simulink model "Formation"  (R2019b)
settings: Solver=FixedStepAuto  StartTime=0.0  StopTime=tf  FixedStep=Ts  RelTol=1e-3
values from neighbouring files (symbols this model uses):
  n = size(L,1)    [Formation_Design.m]    (also in Sim_Parameters.m = 4; anim.m = size(z_tt,1))
  z_0_t = [-2    2    0 ... (first row only)    [Formation_Design.m]
libraries: eeGeneralControl x1
settings Model: Creator=AMIN  LastModifiedBy=AMIN
settings DataIOCC: SaveFormat=Array  ReturnWorkspaceOutputs=off
settings SFSimCC: CustomCodeUndefinedFunction=UseInterfaceOnly

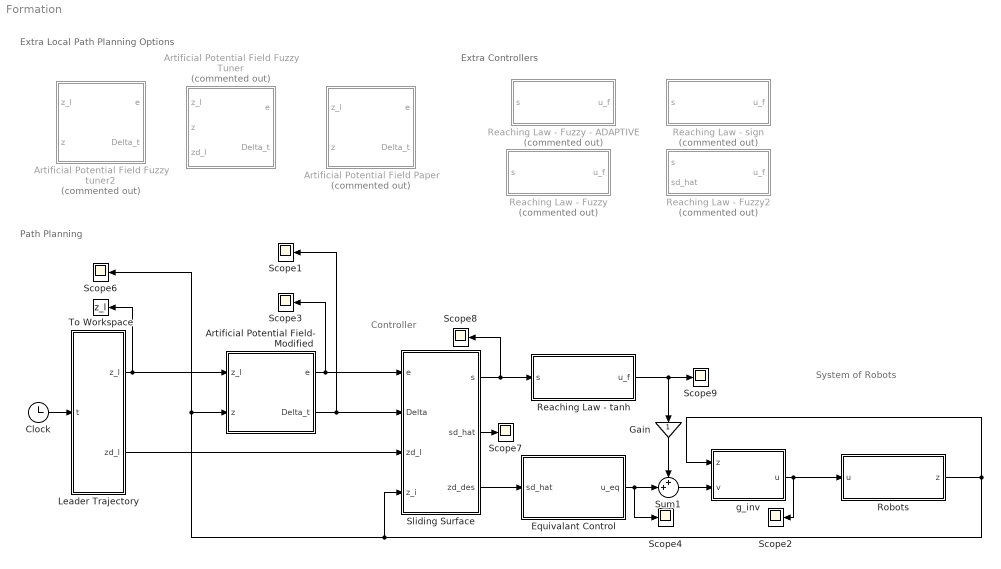
== system Formation ==
  note: Extra Local Path Planning Options
  note: Extra Controllers
  note: System of Robots
  note: Controller
  note: Path Planning
  Artificial Potential Field Fuzzy Tuner : Subsystem  Commented=on
  Artificial Potential Field Fuzzy tuner2 : Subsystem  Commented=on
  Artificial Potential Field Paper : Subsystem  Commented=on
  Artificial Potential Field- Modified : Subsystem
  Clock : Clock
  Equivalant Control : MATLAB Function  TreatAsAtomicUnit=on
  Gain : Gain
  Leader Trajectory : MATLAB Function  TreatAsAtomicUnit=on
  Reaching Law - Fuzzy : Subsystem  Commented=on
  "Reaching Law - Fuzzy - ADAPTIVE " : Subsystem  Commented=on
  Reaching Law - Fuzzy2 : Subsystem  Commented=on
  Reaching Law - sign : Subsystem  Commented=on
  Reaching Law - tanh : Subsystem
  Robots : Subsystem
  Scope{1..4,6..9} (8 alike) : Scope
  Sliding Surface : Subsystem
  Sum1 : Sum  Inputs=++|
  To Workspace : ToWorkspace  VariableName=z_l  SampleTime=-1
  g_inv : MATLAB Function  TreatAsAtomicUnit=on
  wires:
  Sum1/1 -> g_inv/2(v)
  Robots/1(z) -> g_inv/1(z), Sliding Surface/4(z_i), Artificial Potential Field- Modified/2(z), Scope6/1
  Clock/1 -> Leader Trajectory/1(t)
  Leader Trajectory/1(z_l) -> To Workspace/1, Artificial Potential Field- Modified/1(z_l)
  Sliding Surface/1(s) -> Reaching Law - tanh/1(s), Scope8/1
  Equivalant Control/1(u_eq) -> Sum1/2, Scope4/1
  Gain/1 -> Sum1/1
  Leader Trajectory/2(zd_l) -> Sliding Surface/3(zd_l)
  Sliding Surface/3(zd_des) -> Equivalant Control/1(sd_hat)
  Sliding Surface/2(sd_hat) -> Scope7/1
  g_inv/1(u) -> Robots/1(u), Scope2/1
  Artificial Potential Field- Modified/1(e) -> Scope3/1, Sliding Surface/1(e)
  Artificial Potential Field- Modified/2(Delta_t) -> Scope1/1, Sliding Surface/2(Delta)
  Reaching Law - tanh/1(u_f) -> Gain/1, Scope9/1

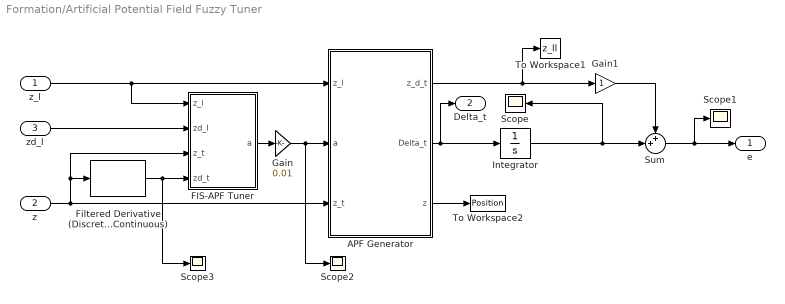
== system Formation/Artificial Potential Field Fuzzy Tuner ==
  z_l : Inport
  z : Inport  Port=2
  zd_l : Inport  Port=3
  APF Generator : MATLAB Function  TreatAsAtomicUnit=on
  FIS-APF Tuner : MATLAB Function  TreatAsAtomicUnit=on
  Filtered Derivative (Discrete or Continuous) : eeGeneralControl/Filtered Derivative (Discrete or Continuous)  K=1  T=100  B=inf  A=-inf  minRatio=10  Ts=-1
      settings: SourceProductName=Simscape Electrical  SourceProductBaseCode=PS
  Gain : Gain  Gain=0.01
  Gain1 : Gain
  Integrator : Integrator
  Scope{,1..3} (4 alike) : Scope
  Sum : Sum  Inputs=++|
  To Workspace1 : ToWorkspace  VariableName=z_ll  SaveFormat=Structure With Time  SampleTime=-1
  To Workspace2 : ToWorkspace  VariableName=Position  SaveFormat=Structure With Time  SampleTime=-1
  e : Outport  VectorParamsAs1DForOutWhenUnconnected=off
  Delta_t : Outport  Port=2  VectorParamsAs1DForOutWhenUnconnected=off
  wires:
  Sum/1 -> e/1, Scope1/1
  APF Generator/1(z_d_t) -> To Workspace1/1, Gain1/1
  Integrator/1 -> Scope/1, Sum/2
  APF Generator/2(Delta_t) -> Integrator/1, Delta_t/1
  Gain1/1 -> Sum/1
  FIS-APF Tuner/1(a) -> Gain/1
  APF Generator/3(z) -> To Workspace2/1
  Gain/1 -> APF Generator/2(a), Scope2/1
  z_l/1 -> FIS-APF Tuner/1(z_l), APF Generator/1(z_l)
  zd_l/1 -> FIS-APF Tuner/2(zd_l)
  z/1 -> APF Generator/3(z_t), Filtered Derivative (Discrete or Continuous)/1, FIS-APF Tuner/3(z_t)
  Filtered Derivative (Discrete or Continuous)/1 -> Scope3/1, FIS-APF Tuner/4(zd_t)

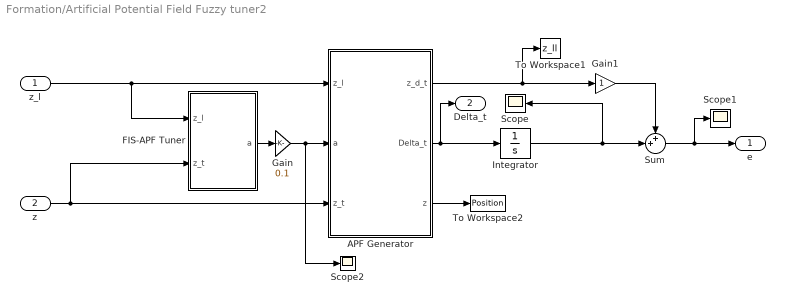
== system Formation/Artificial Potential Field Fuzzy tuner2 ==
  z_l : Inport
  z : Inport  Port=2
  APF Generator : MATLAB Function  TreatAsAtomicUnit=on
  FIS-APF Tuner : MATLAB Function  TreatAsAtomicUnit=on
  Gain : Gain  Gain=0.1
  Gain1 : Gain
  Integrator : Integrator
  Scope : Scope
  Scope1 : Scope
  Scope2 : Scope
  Sum : Sum  Inputs=++|
  To Workspace1 : ToWorkspace  VariableName=z_ll  SaveFormat=Structure With Time  SampleTime=-1
  To Workspace2 : ToWorkspace  VariableName=Position  SaveFormat=Structure With Time  SampleTime=-1
  e : Outport  VectorParamsAs1DForOutWhenUnconnected=off
  Delta_t : Outport  Port=2  VectorParamsAs1DForOutWhenUnconnected=off
  wires:
  Sum/1 -> e/1, Scope1/1
  APF Generator/1(z_d_t) -> To Workspace1/1, Gain1/1
  Integrator/1 -> Scope/1, Sum/2
  APF Generator/2(Delta_t) -> Integrator/1, Delta_t/1
  Gain1/1 -> Sum/1
  FIS-APF Tuner/1(a) -> Gain/1
  APF Generator/3(z) -> To Workspace2/1
  Gain/1 -> APF Generator/2(a), Scope2/1
  z_l/1 -> FIS-APF Tuner/1(z_l), APF Generator/1(z_l)
  z/1 -> APF Generator/3(z_t), FIS-APF Tuner/2(z_t)

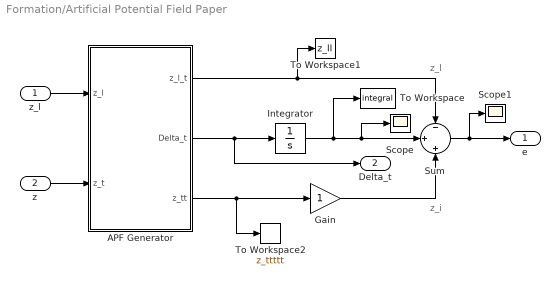
== system Formation/Artificial Potential Field Paper ==
  note: z_l
  note: z_i
  z_l : Inport
  z : Inport  Port=2
  APF Generator : MATLAB Function  TreatAsAtomicUnit=on
  Gain : Gain
  Integrator : Integrator
  Scope : Scope
  Scope1 : Scope
  Sum : Sum  Inputs=-|+|+
  To Workspace : ToWorkspace  VariableName=integral  SaveFormat=Structure With Time  SampleTime=-1
  To Workspace1 : ToWorkspace  VariableName=z_ll  SaveFormat=Structure With Time  SampleTime=-1
  To Workspace2 : ToWorkspace  VariableName=z_ttttt  SaveFormat=Structure With Time  SampleTime=-1
  e : Outport  VectorParamsAs1DForOutWhenUnconnected=off
  Delta_t : Outport  Port=2  VectorParamsAs1DForOutWhenUnconnected=off
  wires:
  APF Generator/2(Delta_t) -> Delta_t/1, Integrator/1
  z_l/1 -> APF Generator/1(z_l)
  z/1 -> APF Generator/2(z_t)
  Integrator/1 -> Scope/1, Sum/2, To Workspace/1
  APF Generator/1(z_l_t) -> To Workspace1/1, Sum/1
  APF Generator/3(z_tt) -> Gain/1, To Workspace2/1
  Sum/1 -> Scope1/1, e/1
  Gain/1 -> Sum/3

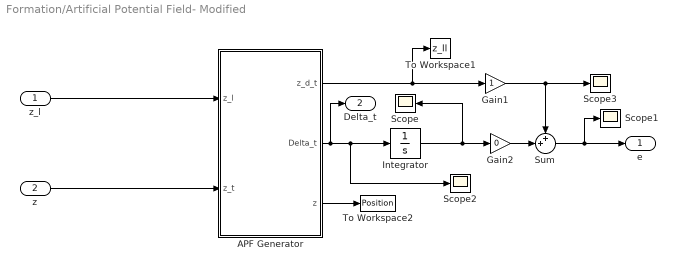
== system Formation/Artificial Potential Field- Modified ==
  z_l : Inport
  z : Inport  Port=2
  APF Generator : MATLAB Function  TreatAsAtomicUnit=on
  Gain1 : Gain
  Gain2 : Gain  Gain=0
  Integrator : Integrator
  Scope{,1..3} (4 alike) : Scope
  Sum : Sum  Inputs=++|
  To Workspace1 : ToWorkspace  VariableName=z_ll  SaveFormat=Structure With Time  SampleTime=-1
  To Workspace2 : ToWorkspace  VariableName=Position  SaveFormat=Structure  SampleTime=-1
  e : Outport  VectorParamsAs1DForOutWhenUnconnected=off
  Delta_t : Outport  Port=2  VectorParamsAs1DForOutWhenUnconnected=off
  wires:
  z/1 -> APF Generator/2(z_t)
  z_l/1 -> APF Generator/1(z_l)
  APF Generator/3(z) -> To Workspace2/1
  Gain1/1 -> Scope3/1, Sum/1
  APF Generator/2(Delta_t) -> Delta_t/1, Scope2/1, Integrator/1
  Integrator/1 -> Gain2/1, Scope/1
  APF Generator/1(z_d_t) -> Gain1/1, To Workspace1/1
  Sum/1 -> Scope1/1, e/1
  Gain2/1 -> Sum/2

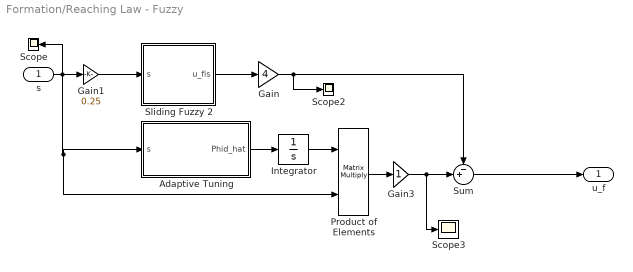
== system Formation/Reaching Law - Fuzzy ==
  s : Inport
  Adaptive Tuning : MATLAB Function  TreatAsAtomicUnit=on
  Gain : Gain  Gain=4
  Gain1 : Gain  Gain=0.25
  Gain3 : Gain
  Integrator : Integrator  InitialCondition=zeros(n)
  Product of Elements : Product  Multiplication=Matrix(*)
  Scope : Scope
  Scope2 : Scope
  Scope3 : Scope
  Sliding Fuzzy 2 : MATLAB Function  TreatAsAtomicUnit=on
  Sum : Sum  Inputs=-+|
  u_f : Outport  VectorParamsAs1DForOutWhenUnconnected=off
  wires:
  Gain/1 -> Scope2/1, Sum/1
  s/1 -> Product of Elements/2, Adaptive Tuning/1(s), Gain1/1, Scope/1
  Sliding Fuzzy 2/1(u_fis) -> Gain/1
  Gain1/1 -> Sliding Fuzzy 2/1(s)
  Sum/1 -> u_f/1
  Adaptive Tuning/1(Phid_hat) -> Integrator/1
  Product of Elements/1 -> Gain3/1
  Gain3/1 -> Sum/2, Scope3/1
  Integrator/1 -> Product of Elements/1

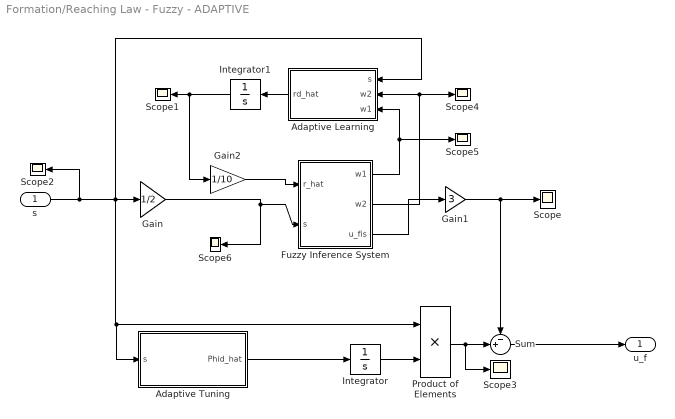
== system Formation/Reaching Law - Fuzzy - ADAPTIVE  ==
  s : Inport
  Adaptive Learning : MATLAB Function  TreatAsAtomicUnit=on
  Adaptive Tuning : MATLAB Function  TreatAsAtomicUnit=on
  Fuzzy Inference System : MATLAB Function  TreatAsAtomicUnit=on
  Gain : Gain  Gain=1/2
  Gain1 : Gain  Gain=3
  Gain2 : Gain  Gain=1/10
  Integrator : Integrator
  Integrator1 : Integrator
  Product of Elements : Product
  Scope{,1..6} (7 alike) : Scope
  Sum : Sum  Inputs=-+|
  u_f : Outport  VectorParamsAs1DForOutWhenUnconnected=off
  wires:
  Sum/1 -> u_f/1
  Adaptive Tuning/1(Phid_hat) -> Integrator/1
  Fuzzy Inference System/3(u_fis) -> Gain1/1
  Adaptive Learning/1(rd_hat) -> Integrator1/1
  Integrator1/1 -> Gain2/1, Scope1/1
  Fuzzy Inference System/1(w1) -> Adaptive Learning/3(w1), Scope5/1
  Integrator/1 -> Product of Elements/2
  Product of Elements/1 -> Scope3/1, Sum/2
  Fuzzy Inference System/2(w2) -> Adaptive Learning/2(w2), Scope4/1
  s/1 -> Scope2/1, Product of Elements/1, Adaptive Tuning/1(s), Gain/1, Adaptive Learning/1(s)
  Gain/1 -> Scope6/1, Fuzzy Inference System/2(s)
  Gain1/1 -> Scope/1, Sum/1
  Gain2/1 -> Fuzzy Inference System/1(r_hat)

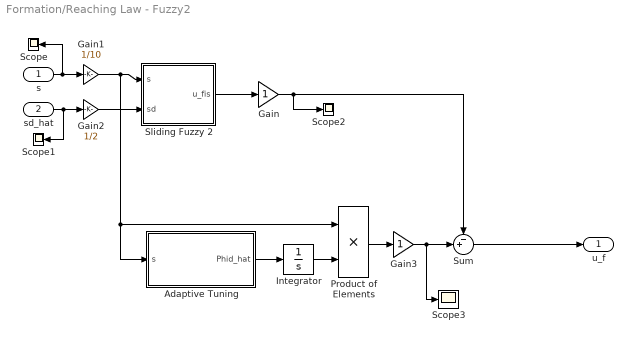
== system Formation/Reaching Law - Fuzzy2 ==
  s : Inport
  sd_hat : Inport  Port=2
  Adaptive Tuning : MATLAB Function  TreatAsAtomicUnit=on
  Gain : Gain
  Gain1 : Gain  Gain=1/10
  Gain2 : Gain  Gain=1/2
  Gain3 : Gain
  Integrator : Integrator
  Product of Elements : Product
  Scope{,1..3} (4 alike) : Scope
  Sliding Fuzzy 2 : MATLAB Function  TreatAsAtomicUnit=on
  Sum : Sum  Inputs=-+|
  u_f : Outport  VectorParamsAs1DForOutWhenUnconnected=off
  wires:
  Gain3/1 -> Scope3/1, Sum/2
  Product of Elements/1 -> Gain3/1
  Adaptive Tuning/1(Phid_hat) -> Integrator/1
  Sum/1 -> u_f/1
  Integrator/1 -> Product of Elements/2
  Gain1/1 -> Adaptive Tuning/1(s), Product of Elements/1, Sliding Fuzzy 2/1(s)
  Sliding Fuzzy 2/1(u_fis) -> Gain/1
  s/1 -> Scope/1, Gain1/1
  Gain/1 -> Sum/1, Scope2/1
  sd_hat/1 -> Scope1/1, Gain2/1
  Gain2/1 -> Sliding Fuzzy 2/2(sd)

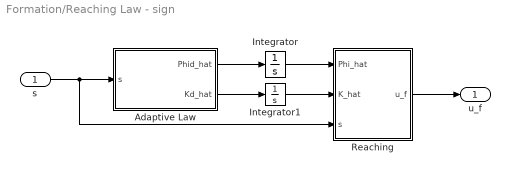
== system Formation/Reaching Law - sign ==
  s : Inport
  Adaptive Law : MATLAB Function  TreatAsAtomicUnit=on
  Integrator : Integrator
  Integrator1 : Integrator
  Reaching : MATLAB Function  TreatAsAtomicUnit=on
  u_f : Outport  VectorParamsAs1DForOutWhenUnconnected=off
  wires:
  Integrator1/1 -> Reaching/2(K_hat)
  Adaptive Law/2(Kd_hat) -> Integrator1/1
  Integrator/1 -> Reaching/1(Phi_hat)
  Adaptive Law/1(Phid_hat) -> Integrator/1
  Reaching/1(u_f) -> u_f/1
  s/1 -> Adaptive Law/1(s), Reaching/3(s)

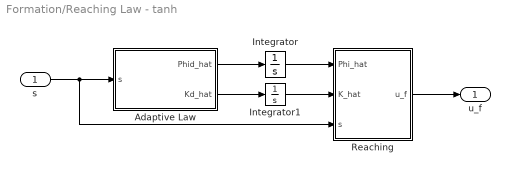
== system Formation/Reaching Law - tanh ==
  s : Inport
  Adaptive Law : MATLAB Function  TreatAsAtomicUnit=on
  Integrator : Integrator
  Integrator1 : Integrator
  Reaching : MATLAB Function  TreatAsAtomicUnit=on
  u_f : Outport  VectorParamsAs1DForOutWhenUnconnected=off
  wires:
  s/1 -> Reaching/3(s), Adaptive Law/1(s)
  Reaching/1(u_f) -> u_f/1
  Adaptive Law/1(Phid_hat) -> Integrator/1
  Integrator/1 -> Reaching/1(Phi_hat)
  Adaptive Law/2(Kd_hat) -> Integrator1/1
  Integrator1/1 -> Reaching/2(K_hat)

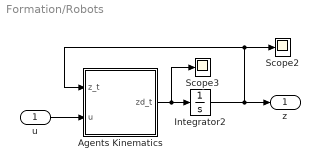
== system Formation/Robots ==
  u : Inport
  Agents Kinematics : MATLAB Function  TreatAsAtomicUnit=on
  Integrator2 : Integrator  InitialCondition=z_0_t
  Scope2 : Scope
  Scope3 : Scope
  z : Outport  VectorParamsAs1DForOutWhenUnconnected=off
  wires:
  u/1 -> Agents Kinematics/2(u)
  Agents Kinematics/1(zd_t) -> Scope3/1, Integrator2/1
  Integrator2/1 -> z/1, Agents Kinematics/1(z_t), Scope2/1

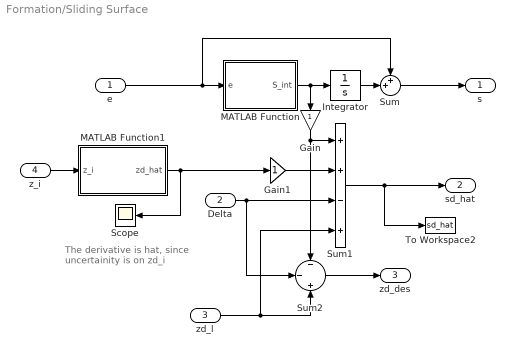
== system Formation/Sliding Surface ==
  note: The derivative is hat,
      | since uncertainity is on zd_i
  e : Inport
  Delta : Inport  Port=2
  zd_l : Inport  Port=3
  z_i : Inport  Port=4
  Gain : Gain
  Gain1 : Gain
  Integrator : Integrator
  MATLAB Function : MATLAB Function  TreatAsAtomicUnit=on
  MATLAB Function1 : MATLAB Function  TreatAsAtomicUnit=on
  Scope : Scope
  Sum : Sum  Inputs=++|
  Sum1 : Sum  Inputs=++-+
  Sum2 : Sum  Inputs=-|-|+
  To Workspace2 : ToWorkspace  VariableName=sd_hat  SampleTime=-1
  s : Outport  VectorParamsAs1DForOutWhenUnconnected=off
  sd_hat : Outport  Port=2  VectorParamsAs1DForOutWhenUnconnected=off
  zd_des : Outport  Port=3  VectorParamsAs1DForOutWhenUnconnected=off
  wires:
  e/1 -> MATLAB Function/1(e), Sum/1
  Integrator/1 -> Sum/2
  MATLAB Function/1(S_int) -> Integrator/1, Gain/1
  Sum/1 -> s/1
  zd_l/1 -> Sum2/3, Sum1/4
  z_i/1 -> MATLAB Function1/1(z_i)
  MATLAB Function1/1(zd_hat) -> Scope/1, Gain1/1
  Gain/1 -> Sum2/1, Sum1/1
  Sum2/1 -> zd_des/1
  Delta/1 -> Sum1/3, Sum2/2
  Gain1/1 -> Sum1/2
  Sum1/1 -> sd_hat/1, To Workspace2/1

== matlab function Formation/Artificial Potential Field Paper/APF Generator ==
  data: z_l_t output; Delta_t output; z_l input; z_t input; z_tt output
function [z_l_t,Delta_t,z_tt] =  APF(z_l,z_t)

z_tt = z_t(:,1:2); %excluding orientation
n = size(z_t,1);
Delta_l = zeros(n,2);
Delta_i = zeros(n,2);

%% Field Gradian Calculatoin & Sum
% Inter-agent field interactions 
    for i=1:1:n
        for j=1:1:n
            Delta_i(i,:) = Potential_Function(z_tt(i,:),z_tt(j,:));
        end
    end

    % Leader - agent interaction
    for i=1:1:n
        Delta_l(i,:) = Potential_Function(z_tt(i,:),z_l.');
    end
    
    Delta_t = Delta_l + Delta_i;
    
    %% Generalizing the Z_l for everyone
    z_l_t = zeros(n,2);
    for i=1:1:n
        z_l_t(i,:) = z_l.';
    end

end

== matlab function Formation/Sliding Surface/MATLAB Function ==
  data: e input; S_int output
function S_int = fcn(e)
[n,~,~,~,beta,~,~,~,~,~,lambda1,lambda2]= Sim_Parameters();
%n = size(e,1);
S_int = zeros(n,2);


    for i=1:1:n
        A = (abs(e(i,:)).^(1+1/beta)).';
        B = (abs(e(i,:)).^(1-1/beta)).';
        S_int(i,:) = (lambda1*eye(2)*(A.*sign(e(i,:)).')+lambda2*eye(2)*(B.*sign(e(i,:)).')).';
    end
    
end

== matlab function Formation/Leader Trajectory ==
  data: z_l output; t input; zd_l output
function [z_l,zd_l] =  TRJ(t)
[n,~]= Sim_Parameters();
[~,z_0_l,~,~]= Formation_Design();
%% Moving
% Sin in y direction
% z_l = 1*[z_0_l(1)+0.1*t ;z_0_l(2)+1*sin(0.1*t)];
% zd =1* [0.1;0.1*cos(0.1*t)];

% Circle
% z_l =[z_0_l(1)+2*sin(0.1*t) ; z_0_l(2)+2*cos(0.1*t)];
% zd =[0.2*cos(0.01*t);-0.2*sin(0.01*t)];

% Line
% z_l = 1*[z_0_l(1)+0.1*t ;z_0_l(2)];
% zd =1* [0.1;0];

%% Static
z_l =[z_0_l(1) ; z_0_l(2)];
zd =[0;0];

zd_l = zeros(n,2);
    for i=1:1:n
        zd_l(i,:) = zd.';
    end

end

== matlab function Formation/Reaching Law - tanh/Reaching ==
  data: Phi_hat input; K_hat input; s input; u_f output
function u_f = RL(Phi_hat,K_hat,s)

    u_f = -K_hat*tanh(0.01*s)-Phi_hat*s ;
    
end

== matlab function Formation/Equivalant Control ==
  data: u_eq output; sd_hat input
function u_eq =  estimator(sd_hat)
    u_eq = sd_hat;                 % perfect tracking
end

== matlab function Formation/g_inv ==
  data: z input; u output; v input
function u =  g_inv(z,v)
    u = v;              % for easy dimentioning
    n = size(z,1);
    q_t = z(:,3);     % extracting qs from states

    for i=1:1:n
        L = 0.21;
        g = [ cos(q_t(i)) -L*sin(q_t(i));
              sin(q_t(i))  L*cos(q_t(i))];

        u(i,:) = (inv(g)*v(i,:).').';
    end
end

== matlab function Formation/Robots/Agents Kinematics ==
  settings: updateMethod=DISCRETE
  data: z_t input; zd_t output; u input
function zd_t  = KIN(z_t,u)

    n = size(u,1);
    zd_t =zeros(n,3);
    d = 1*[0.01;0.01];                  % The lumped uncertainity
    
   for i=1:1:n
        
        [zd_t(i,1:2),zd_t(i,3)] = Agent_Kinematics(z_t(i,3),u(i,:),d);
        
    end 

end

== matlab function Formation/Reaching Law - tanh/Adaptive Law ==
  data: Phid_hat output; Kd_hat output; s input
function [Phid_hat,Kd_hat] = ADP(s)
    [~,~,~,~,~,delta,gamma,~,~,~,~,~]= Sim_Parameters();
    miu = 1;
    Kd_hat = (1/delta)*tanh(miu*s)*s.';
    Phid_hat = (1/gamma)*(s*s.');
end

== matlab function Formation/Sliding Surface/MATLAB Function1 ==
  data: z_i input; zd_hat output
function zd_hat = RefMDL(z_i)
%     [n,~]= Sim_Parameters();
%     q = z_i(1,3);
%     %n = size(z_i,1);
%     zd_hat = zeros(n,2);
%     d = 0;
%     
%     for i=1:1:n
%         
%         [zd_hat(i,1:2),~] = Agent_Kinematics(q(i),z_i(i,1:2),d);
%         
%     end 
         
 
    zd_hat = 0;
end

== matlab function Formation/Reaching Law - Fuzzy - ADAPTIVE /Adaptive Tuning ==
  data: s input; Phid_hat output
function Phid_hat = ADT(s)
[~,~,~,~,~,~,gamma,~,~,~,~,~]= Sim_Parameters();
%% Adaptive Law
Phid_hat = (1/gamma)*(s*s.');
end

== matlab function Formation/Reaching Law - Fuzzy - ADAPTIVE /Adaptive Learning ==
  data: s input; w2 input; rd_hat output; w1 input
function rd_hat = fcn(s,w2,w1)
[~,~,~,alpha,~,~,~,~,~,~,~,~]= Sim_Parameters();
%% Adaptive Law
rd_hat = (1/alpha)*(w1-w2)*s.';
end

== matlab function Formation/Reaching Law - Fuzzy - ADAPTIVE /Fuzzy Inference System ==
  data: r_hat input; w1 output; w2 output; s input; u_fis output
function [w1,w2,u_fis] = FIS(r_hat,s)
%% Decomposition of Signals
n = size(s,1);
w1 = zeros(n,2);
w2 = zeros(n,2);
u_fis = zeros(n,2);
%% Constuction of Fuzzy Structure
% input = struct();
% output = struct();
% rule = struct();
% FIS = struct('name','Slide_FIS','type','mamdani','andMethod','min','orMethod','max','defuzzMethod','centroid','impMethod','min','aggMethod','max','input',,'output',,'rule',);
%% 2*n Fuzzy Systems
% Each Agent has 2 fuzzy systems, for x and y and their parameters are
% adaptive.

    for i=1:1:n            % Agent Indexing
        for j=1:1:2        % X & Y Indexing         
            %% FUZZY LOAD AND DEPOLY
            Gain = 1;
            ss = Gain*s(i,j);
            FIS = getFISCodeGenerationData('Sliding_FIS');

            [~,~,~,~,ruleFiring] = evalfis(FIS,ss); % Fuzzy Computaion
            u_fis(i,j) = evalfis(FIS,ss);     % Fuzzy Output
            w1(i,j) = ruleFiring(3) ;      % PE rule  Fire Strength
            w2(i,j) = ruleFiring(1) ;      % NE rule  Fire Strength
            %FIS.output.mf(1).params = [-2-r_hat(i,j) -1-r_hat(i,j) -r_hat(i,j)]; % Shifting Output
            %FIS.output.mf(3).params = [r_hat(i,j) 1+r_hat(i,j) 2-r_hat(i,j)]; % Shifting Output
            
        end
    end
    
end

== matlab function Formation/Reaching Law - Fuzzy/Sliding Fuzzy 2 ==
  data: s input; u_fis output
function u_fis = fcn(s)
%% Decomposition of Signals
[n,~]= Sim_Parameters();
%n = size(s,1);
u_fis = zeros(n,2);
%% 2*n Fuzzy Systems
% Each Agent has 2 fuzzy systems, for x and y and their parameters are
% adaptive.

    for i=1:1:n            % Agent Indexing
        for j=1:1:2        % X & Y Indexing         
            %% FUZZY LOAD AND DEPOLY
            ss = s(i,j);
            FIS = getFISCodeGenerationData('Sliding_FIS');
            u_fis(i,j) = evalfis(FIS,ss);     % Fuzzy Output                        
        end
    end
end

== matlab function Formation/Reaching Law - Fuzzy/Adaptive Tuning ==
  data: s input; Phid_hat output
function Phid_hat = ADT(s)
[n,~,~,~,~,~,gamma,~,~,~,~,~]= Sim_Parameters();
%% Adaptive Law
Phid_hat = zeros(n);
Phid_hat = (1/gamma)*(s*s.');
end

== matlab function Formation/Reaching Law - Fuzzy2/Adaptive Tuning ==
  data: s input; Phid_hat output
function Phid_hat = ADT(s)
[~,~,~,~,~,~,gamma,~,~,~,~,~]= Sim_Parameters();
%% Adaptive Law
Phid_hat = (1/500)*(s*s.');
end

== matlab function Formation/Reaching Law - Fuzzy2/Sliding Fuzzy 2 ==
  data: s input; u_fis output; sd input
function u_fis = fcn(s,sd)
%% Decomposition of Signals
n = size(s,1);
u_fis = zeros(n,2);
%% 2*n Fuzzy Systems
% Each Agent has 2 fuzzy systems, for x and y and their parameters are
% adaptive.

    for i=1:1:n            % Agent Indexing
        for j=1:1:2        % X & Y Indexing         
            %% FUZZY LOAD AND DEPOLY
            ss = [s(i,j);sd(i,j)];
            FIS = getFISCodeGenerationData('Sliding_FIS2');
            u_fis(i,j) = evalfis(FIS,ss);     % Fuzzy Output                        
        end
    end
end

== matlab function Formation/Reaching Law - sign/Adaptive Law ==
  data: Phid_hat output; Kd_hat output; s input
function [Phid_hat,Kd_hat] = ADP(s)
    [~,~,~,~,~,delta,gamma,~,~,~,~,~]= Sim_Parameters();
    miu = 1;
    Kd_hat = (1/delta)*tanh(miu*s)*s.';
    Phid_hat = (1/gamma)*(s*s.');
end

== matlab function Formation/Reaching Law - sign/Reaching ==
  data: Phi_hat input; K_hat input; s input; u_f output
function u_f = RL(Phi_hat,K_hat,s)

    u_f = -K_hat*sign(s)-Phi_hat*s ;
    
end

== matlab function Formation/Artificial Potential Field Fuzzy Tuner/APF Generator ==
  data: z_d_t output; Delta_t output; z_l input; a input; z_t input; z output
function [z_d_t,Delta_t,z] =  APF(z_l,a,z_t)
[n,~]= Sim_Parameters();
[~,~,L,z_rf]= Formation_Design();

z = z_t(:,1:2); %excluding orientation
moment = zeros(n,2);
Delta_l = zeros(n,2);
Delta_i = zeros(n,2);
z_d_t = zeros(n,2);
%% Field Grad Calculatoin & Sum
    % Inter-agent field interactions 
    for i=1:1:n
        for j=1:1:n
            Delta_i(i,:) = Potential_Function2(z(i,:),z(j,:),z_rf{i,j},L(i,j),a(i,j));
            
        end
    end

    % Leader - Agent Interaction
    for i=1:1:n
        Delta_l(i,:) = Potential_Function2(z(i,:),z_l.',z_rf{i,n+1},L(i,n+1),a(i,n+1));
    end
    
    Delta_t = Delta_l + Delta_i;
    
    %% Generalizing the Z_l for everyone
    z_l_t = zeros(n,2);
    for i=1:1:n
        z_l_t(i,:) = z_l.';
    end
    %% Part one of error signal
%     for i=1:1:n
%         for j=1:1:n
%             if L(i,n+1) == 0
%             z_d_t(i,:) = z_d_t(i,:) - L(i,j)*z(j,:);
%             end
%         end
%         z_d_t(i,:) = z(i,:)- z_d_t(i,:) - L(i,n+1)*z_l_t(i,:);
%     end
           z_d_t(1,:) = 1*(z(1,:) - z_l.' - z_rf{1,5});
           z_d_t(2,:) = 1*(z(2,:) - z_l.' - z_rf{2,5});
           z_d_t(3,:) = 1*(z(3,:) - z(1,:)- z_rf{3,1});
           z_d_t(4,:) = 1*(z(4,:) - z(2,:)- z_rf{4,2});
end

== matlab function Formation/Artificial Potential Field Fuzzy Tuner/FIS-APF Tuner ==
  data: z_l input; zd_l input; z_t input; a output; zd_t input
function a = fcn(z_l,zd_l,z_t,zd_t)
    [z_0_t,~,L,z_rf]= Formation_Design();
    n = size(z_0_t,1);
    z = z_t(:,1:2); %excluding orientation
    zd = zd_t(:,1:2); %excluding orientation
    %% Parameter Update for Attraction
    % All the attractions among agents and leader-agents updates here via
    % the FIS.
    a = zeros(n+1);
    ig =1/5;            %inputgain for distance
    for i=1:1:n
        for j=1:1:n
            if L(i,j)== 1
                 d = z(i,:) - z(j,:)+z_rf{i,j};
                 dis =ig*norm(d);
                 d_dot = zd(i,:) - zd(j,:);
                 ddis = norm(d_dot)*sign(sign(d_dot(1))+sign(d_dot(2))-1);
                 %% Deploy Fuzzy
                 FIS = getFISCodeGenerationData('Att_FIS');
                 a(i,j) = evalfis(FIS,[dis ddis]);       % Fuzzy Output
                 
            end
        end
        
        if L(i,n+1) == 1
                 d = z(i,:) - z_l.'+z_rf{i,n+1};
                 dis = ig*norm(d);
                 d_dot = zd(i,:) - zd_l(i,:);
                 ddis = norm(d_dot)*sign(d_dot(1)+d_dot(2)-1);
                 %% Deploy Fuzzy
                 %FIS = getFISCodeGenerationData('Att_FIS');
                 a(i,n+1) = evalfis(FIS,[dis ddis]);        % Fuzzy Output
        end

    end
end

== matlab function Formation/Artificial Potential Field- Modified/APF Generator ==
  data: z_d_t output; Delta_t output; z_l input; z_t input; z output
function [z_d_t,Delta_t,z] =  APF(z_l,z_t)
[n,~]= Sim_Parameters();
[~,~,L,z_rf]= Formation_Design();

z = z_t(:,1:2); %excluding orientation
%moment = zeros(n,2);
Delta_l = zeros(n,2);
Delta_i = zeros(n,2);
z_d_t = zeros(n,2);
%% Field Grad Calculatoin & Sum
    % Inter-agent field interactions 
    for i=1:1:n
        for j=1:1:n
            Delta_i(i,:) = Potential_Function2(z(i,:),z(j,:),z_rf{i,j},L(i,j));
            
        end
    end

    % Leader - Agent Interaction
    for i=1:1:n
        Delta_l(i,:) = Potential_Function2(z(i,:),z_l.',z_rf{i,n+1},L(i,n+1));
    end
    
    Delta_t = Delta_l + Delta_i;
    
    %% Generalizing the Z_l for everyone
    z_l_t = zeros(n,2);
    for i=1:1:n
        z_l_t(i,:) = z_l.';
    end
    %% Part one of error signal
%     for i=1:1:n
%         for j=1:1:n
%             if L(i,n+1) == 0
%             z_d_t(i,:) = z_d_t(i,:) - L(i,j)*z(j,:);
%             end
%         end
%         z_d_t(i,:) = z(i,:)- z_d_t(i,:) - L(i,n+1)*z_l_t(i,:);
%     end
           z_d_t(1,:) = 1*(z(1,:) - z_l.' - z_rf{1,5});
           z_d_t(2,:) = 1*(z(2,:) - z_l.' - z_rf{2,5});
           z_d_t(3,:) = 1*(z(3,:) - z(1,:)- z_rf{3,1});
           z_d_t(4,:) = 1*(z(4,:) - z(2,:)- z_rf{4,2});
end

== matlab function Formation/Artificial Potential Field Fuzzy tuner2/APF Generator ==
  data: z_d_t output; Delta_t output; z_l input; a input; z_t input; z output
function [z_d_t,Delta_t,z] =  APF(z_l,a,z_t)
[n,~]= Sim_Parameters();
[~,~,L,z_rf]= Formation_Design();

z = z_t(:,1:2); %excluding orientation
%moment = zeros(n,2);
Delta_l = zeros(n,2);
Delta_i = zeros(n,2);
z_d_t = zeros(n,2);
%% Field Grad Calculatoin & Sum
    % Inter-agent field interactions 
    for i=1:1:n
        for j=1:1:n
            Delta_i(i,:) = Potential_Function2(z(i,:),z(j,:),z_rf{i,j},L(i,j),a(i,j));
            
        end
    end

    % Leader - Agent Interaction
    for i=1:1:n
        Delta_l(i,:) = Potential_Function2(z(i,:),z_l.',z_rf{i,n+1},L(i,n+1),a(i,n+1));
    end
    
    Delta_t = Delta_l + Delta_i;
    
    %% Generalizing the Z_l for everyone
    z_l_t = zeros(n,2);
    for i=1:1:n
        z_l_t(i,:) = z_l.';
    end
    %% Part one of error signal
%     for i=1:1:n
%         for j=1:1:n
%             if L(i,n+1) == 0
%             z_d_t(i,:) = z_d_t(i,:) - L(i,j)*z(j,:);
%             end
%         end
%         z_d_t(i,:) = z(i,:)- z_d_t(i,:) - L(i,n+1)*z_l_t(i,:);
%     end
           z_d_t(1,:) = 1*(z(1,:) - z_l.' - z_rf{1,5});
           z_d_t(2,:) = 1*(z(2,:) - z_l.' - z_rf{2,5});
           z_d_t(3,:) = 1*(z(3,:) - z(1,:)- z_rf{3,1});
           z_d_t(4,:) = 1*(z(4,:) - z(2,:)- z_rf{4,2});
end

== matlab function Formation/Artificial Potential Field Fuzzy tuner2/FIS-APF Tuner ==
  data: z_l input; z_t input; a output
function a = fcn(z_l,z_t)
    [z_0_t,~,L,z_rf]= Formation_Design();
    n = size(z_0_t,1);
    z = z_t(:,1:2); %excluding orientation
    
    %% Parameter Update for Attraction
    % All the attractions among agents and leader-agents updates here via
    % the FIS.
    a = zeros(n+1);
    ig =1/3;            %inputgain for distance
    for i=1:1:n
        for j=1:1:n
            if L(i,j)== 1
                 d = z(i,:) - z(j,:)+z_rf{i,j};
                 dis =ig*norm(d);
                 %% Deploy Fuzzy
                 FIS = getFISCodeGenerationData('Att_FIS_V2');
                 a(i,j) = evalfis(FIS,dis);       % Fuzzy Output
                 
            end
        end
        
        if L(i,n+1) == 1
                 d = z(i,:) - z_l.'+z_rf{i,n+1};
                 dis = ig*norm(d);
                 %% Deploy Fuzzy
                 %FIS = getFISCodeGenerationData('Att_FIS');
                 a(i,n+1) = evalfis(FIS,dis);        % Fuzzy Output
        end

    end
end
